simulink model "MiMonza"  (R2023b)
settings: Solver=VariableStepAuto  StartTime=0.0  StopTime=20  MaxStep=0.05
libraries: slpidlib x1
settings Model: Creator=Usuario  LastModifiedBy=Usuario
settings SolverCC: ZeroCrossAlgorithm=Adaptive

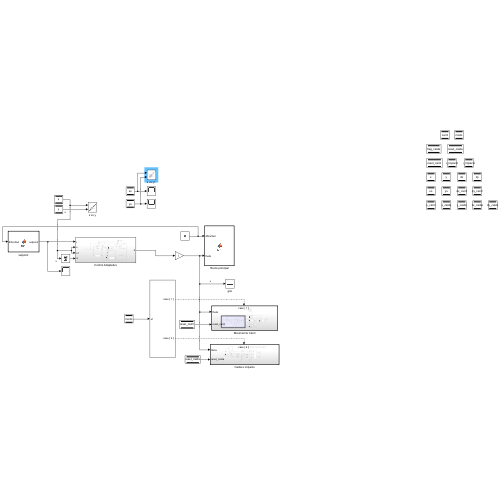
[thumbnail: Simulink's stored preview of the top-level diagram]
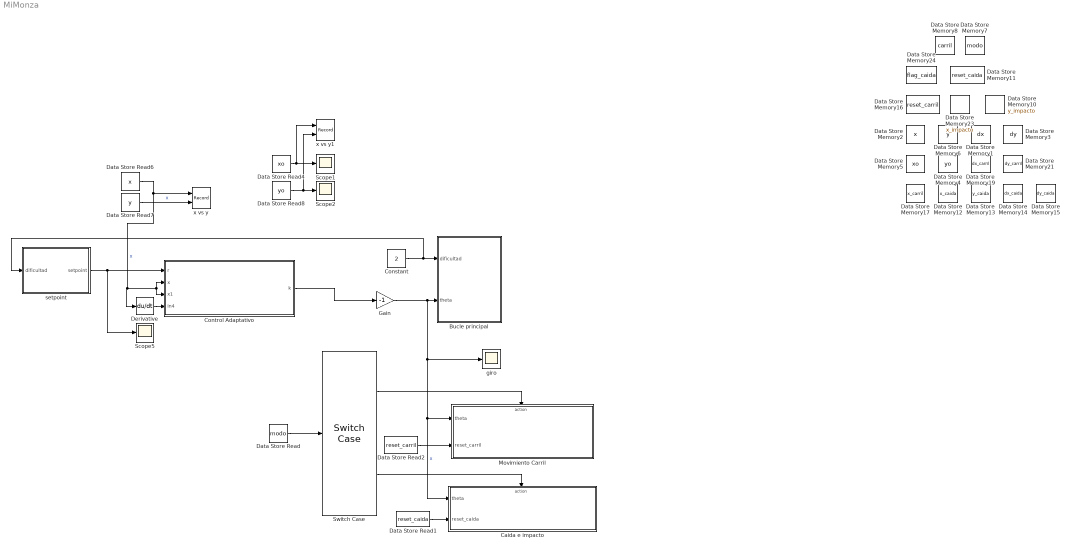
== system MiMonza ==
  " Bucle principal" : MATLAB Function  TreatAsAtomicUnit=on
  Caida e impacto : Subsystem  TreatAsAtomicUnit=on
  Constant : Constant  Value=2
  Control Adaptativo : Subsystem
  Data Store Memory1 : DataStoreMemory  DataStoreName=dx  ReadBeforeWriteMsg=warning  WriteAfterWriteMsg=warning  WriteAfterReadMsg=warning  ShowAdditionalParam=off  OutDataTypeStr=double
  Data Store Memory10 : DataStoreMemory  DataStoreName=y_impacto  ReadBeforeWriteMsg=warning  WriteAfterWriteMsg=warning  WriteAfterReadMsg=warning  ShowAdditionalParam=off  OutDataTypeStr=double
  Data Store Memory11 : DataStoreMemory  DataStoreName=reset_caida  ReadBeforeWriteMsg=warning  WriteAfterWriteMsg=warning  WriteAfterReadMsg=warning  ShowAdditionalParam=off  OutDataTypeStr=double
  Data Store Memory12 : DataStoreMemory  DataStoreName=x_caida  ReadBeforeWriteMsg=warning  WriteAfterWriteMsg=warning  WriteAfterReadMsg=warning  ShowAdditionalParam=off  OutDataTypeStr=double
  Data Store Memory13 : DataStoreMemory  DataStoreName=y_caida  ReadBeforeWriteMsg=warning  WriteAfterWriteMsg=warning  WriteAfterReadMsg=warning  ShowAdditionalParam=off  OutDataTypeStr=double
  Data Store Memory14 : DataStoreMemory  DataStoreName=dx_caida  ReadBeforeWriteMsg=warning  WriteAfterWriteMsg=warning  WriteAfterReadMsg=warning  ShowAdditionalParam=off  OutDataTypeStr=double
  Data Store Memory15 : DataStoreMemory  DataStoreName=dy_caida  ReadBeforeWriteMsg=warning  WriteAfterWriteMsg=warning  WriteAfterReadMsg=warning  ShowAdditionalParam=off  OutDataTypeStr=double
  Data Store Memory16 : DataStoreMemory  DataStoreName=reset_carril  ReadBeforeWriteMsg=warning  WriteAfterWriteMsg=warning  WriteAfterReadMsg=warning  ShowAdditionalParam=off  OutDataTypeStr=double
  Data Store Memory17 : DataStoreMemory  DataStoreName=x_carril  ReadBeforeWriteMsg=warning  WriteAfterWriteMsg=warning  WriteAfterReadMsg=warning  InitialValue=-0.11  ShowAdditionalParam=off  OutDataTypeStr=double
  Data Store Memory19 : DataStoreMemory  DataStoreName=dx_carril  ReadBeforeWriteMsg=warning  WriteAfterWriteMsg=warning  WriteAfterReadMsg=warning  ShowAdditionalParam=off  OutDataTypeStr=double
  Data Store Memory2 : DataStoreMemory  DataStoreName=x  ReadBeforeWriteMsg=warning  WriteAfterWriteMsg=warning  WriteAfterReadMsg=warning  InitialValue=-0.11  ShowAdditionalParam=off  OutDataTypeStr=double
  Data Store Memory21 : DataStoreMemory  DataStoreName=dy_carril  ReadBeforeWriteMsg=warning  WriteAfterWriteMsg=warning  WriteAfterReadMsg=warning  ShowAdditionalParam=off  OutDataTypeStr=double
  Data Store Memory23 : DataStoreMemory  DataStoreName=x_impacto  ReadBeforeWriteMsg=warning  WriteAfterWriteMsg=warning  WriteAfterReadMsg=warning  ShowAdditionalParam=off  OutDataTypeStr=double
  Data Store Memory24 : DataStoreMemory  DataStoreName=flag_caida  ReadBeforeWriteMsg=warning  WriteAfterWriteMsg=warning  WriteAfterReadMsg=warning  ShowAdditionalParam=off  OutDataTypeStr=double
  Data Store Memory3 : DataStoreMemory  DataStoreName=dy  ReadBeforeWriteMsg=warning  WriteAfterWriteMsg=warning  WriteAfterReadMsg=warning  ShowAdditionalParam=off  OutDataTypeStr=double
  Data Store Memory4 : DataStoreMemory  DataStoreName=yo  ReadBeforeWriteMsg=warning  WriteAfterWriteMsg=warning  WriteAfterReadMsg=warning  InitialValue=0.1092  ShowAdditionalParam=off  OutDataTypeStr=double
  Data Store Memory5 : DataStoreMemory  DataStoreName=xo  ReadBeforeWriteMsg=warning  WriteAfterWriteMsg=warning  WriteAfterReadMsg=warning  InitialValue=-0.1  ShowAdditionalParam=off  OutDataTypeStr=double
  Data Store Memory6 : DataStoreMemory  DataStoreName=y  ReadBeforeWriteMsg=warning  WriteAfterWriteMsg=warning  WriteAfterReadMsg=warning  InitialValue=0.106  ShowAdditionalParam=off  OutDataTypeStr=double
  Data Store Memory7 : DataStoreMemory  DataStoreName=modo  ReadBeforeWriteMsg=warning  WriteAfterWriteMsg=warning  WriteAfterReadMsg=warning  InitialValue=1  ShowAdditionalParam=off  OutDataTypeStr=double
  Data Store Memory8 : DataStoreMemory  DataStoreName=carril  ReadBeforeWriteMsg=warning  WriteAfterWriteMsg=warning  WriteAfterReadMsg=warning  InitialValue=1  ShowAdditionalParam=off  OutDataTypeStr=double
  Data Store Read : DataStoreRead  DataStoreName=modo  IndexOptions=Index vector (dialog)  Indices=1  OutputSizes=1
  Data Store Read1 : DataStoreRead  DataStoreName=reset_caida  IndexOptions=Index vector (dialog)  Indices=1  OutputSizes=1
  Data Store Read2 : DataStoreRead  DataStoreName=reset_carril  IndexOptions=Index vector (dialog)  Indices=1  OutputSizes=1
  Data Store Read4 : DataStoreRead  DataStoreName=xo  IndexOptions=Index vector (dialog)  Indices=1  OutputSizes=1
  Data Store Read6 : DataStoreRead  DataStoreName=x  IndexOptions=Index vector (dialog)  Indices=1  OutputSizes=1
  Data Store Read7 : DataStoreRead  DataStoreName=y  IndexOptions=Index vector (dialog)  Indices=1  OutputSizes=1
  Data Store Read8 : DataStoreRead  DataStoreName=yo  IndexOptions=Index vector (dialog)  Indices=1  OutputSizes=1
  Derivative : Derivative
  Gain : Gain  Gain=-1
  Movimiento Carril : Subsystem  TreatAsAtomicUnit=on
  Scope1 : Scope
  Scope2 : Scope
  Scope5 : Scope
  Switch Case : SwitchCase  CaseConditions={1,2}  ShowDefaultCase=off
  giro : Scope
  setpoint : MATLAB Function  TreatAsAtomicUnit=on
  x vs y : Record  FileSettingsInternal="{\"entries\":[{\"content\":{\"excelSettings\":{\"content\":{},\"type\":\"Streamout.ExcelSettings\"}},\"type\":\"Streamout.FileSettingStorage\",\"uuid\":\"\"}],\"packageUris\":[\"http:\\/\\/schema.mathworks.com\\/mf0\\/streamout_blocks\\/R2020a\"],\"version\":\"1.0\"}"  Layout=[1 1]  SignalsInternal="{\"entries\":[{\"content\":{\"signals\":[{\"content\":{\"blockPath\":[],\"dimensions\":[1],\"domain\":\"\",\"lineColor\":\"#a2142f\",\"plots\":[1],\"port\":1,\"sid\":[\"\"],\"signalID\":25020,\"signalName\":\"x\"},\"type\":\"RecordBlkView.Signal\",\"uuid\":\"\"},{\"content\":{\"blockPath\":[],\"dimensions\":[1],\"domain\":\"\",\"lineColor\":\"#139fff\",\"plots\":[1],\"port\":2,\"sid\":[\"\"],\"signalID\":25024,\"signalName\":\"x\"},\"type\":\"RecordBlkView.Signal\",\"uuid\":\"\"}]},\"type\":\"RecordBlkView.InputSignals\",\"uuid\":\"\"}],\"packageUris\":[\"http:\\/\\/schema.mathworks.com\\/mf0\\/streamout_blocks\\/R2020a\"],\"version\":\"1.0\"}"  VisualizationBindings="{\"xyplotplugin\":{\"info\":[{\"series\":[{\"bindingParametersList\":[{\"parameter\":\"X-Axis\",\"signalID\":25020,\"signalName\":\"x\"},{\"parameter\":\"Y-Axis\",\"signalID\":25024,\"signalName\":\"x\"}],\"seriesID\":13625}],\"subplotID\":1}]}}"  CompatibilityTag=XY  st=-1
  x vs y1 : Record  FileSettingsInternal="{\"entries\":[{\"content\":{\"excelSettings\":{\"content\":{},\"type\":\"Streamout.ExcelSettings\"}},\"type\":\"Streamout.FileSettingStorage\",\"uuid\":\"\"}],\"packageUris\":[\"http:\\/\\/schema.mathworks.com\\/mf0\\/streamout_blocks\\/R2020a\"],\"version\":\"1.0\"}"  Layout=[1 1]  SignalsInternal="{\"entries\":[{\"content\":{\"signals\":[{\"content\":{\"blockPath\":[],\"dimensions\":[1],\"domain\":\"\",\"lineColor\":\"#a2142f\",\"plots\":[1],\"port\":1,\"sid\":[\"\"],\"signalID\":25028,\"signalName\":\"Data Store\\nRead4\"},\"type\":\"RecordBlkView.Signal\",\"uuid\":\"\"},{\"content\":{\"blockPath\":[],\"dimensions\":[1],\"domain\":\"\",\"lineColor\":\"#139fff\",\"plots\":[1],\"port\":2,\"sid\":[\"\"],\"signalID\":25032,\"signalName\":\"Data Store\\nRead8\"},\"type\":\"RecordBlkView.Signal\",\"uuid\":\"\"}]},\"type\":\"RecordBlkView.InputSignals\",\"uuid\":\"\"}],\"packageUris\":[\"http:\\/\\/schema.mathworks.com\\/mf0\\/streamout_blocks\\/R2020a\"],\"version\":\"1.0\"}"  VisualizationBindings="{\"xyplotplugin\":{\"info\":[{\"series\":[{\"bindingParametersList\":[{\"parameter\":\"X-Axis\",\"signalID\":25028,\"signalName\":\"Data Store\\nRead4\"},{\"parameter\":\"Y-Axis\",\"signalID\":25032,\"signalName\":\"Data Store\\nRead8\"}],\"seriesID\":36668}],\"subplotID\":1}]}}"  CompatibilityTag=XY  st=-1
  wires:
  Data Store Read2/1 -> Movimiento Carril/2(reset_carril)
  Data Store Read4/1 -> x vs y1/1, Scope1/1
  Data Store Read6/1 -> Derivative/1, Control Adaptativo/2(x), Control Adaptativo/3(x1), x vs y/1  "x"
  Data Store Read/1 -> Switch Case/1
  Gain/1 -> " Bucle principal"/2(theta), Caida e impacto/1(theta), Movimiento Carril/1(theta), giro/1  "x"
  Data Store Read7/1 -> x vs y/2  "x"
  Switch Case/1 -> Movimiento Carril/Action
  Constant/1 -> setpoint/1(dificultad), " Bucle principal"/1(dificultad)
  Data Store Read8/1 -> x vs y1/2, Scope2/1
  setpoint/1(setpoint) -> Control Adaptativo/1(r), Scope5/1
  Switch Case/2 -> Caida e impacto/Action
  Data Store Read1/1 -> Caida e impacto/2(reset_caida)
  Derivative/1 -> Control Adaptativo/4(In4)
  Control Adaptativo/1(k) -> Gain/1

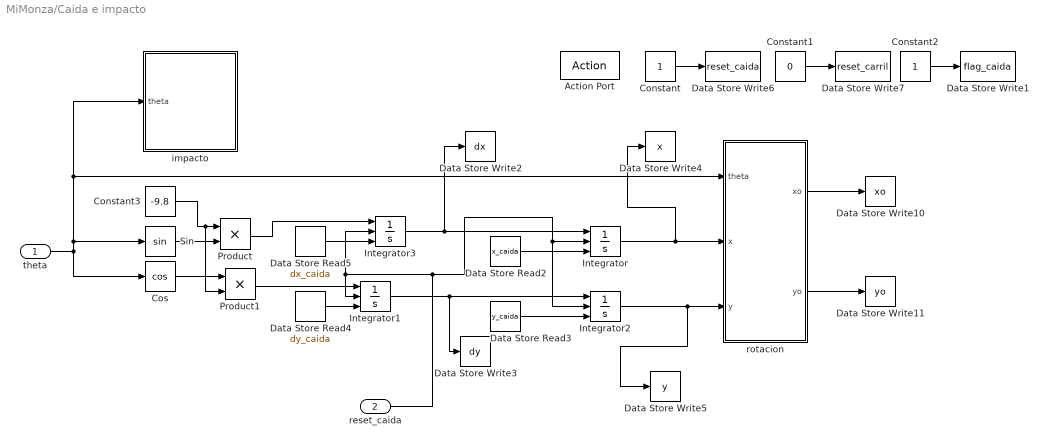
== system MiMonza/Caida e impacto ==
  theta : Inport
  reset_caida : Inport  Port=2
  Action Port : ActionPort  ActionPortLabel=case [ 2 ]:
  Constant : Constant
  Constant1 : Constant  Value=0
  Constant2 : Constant
  Constant3 : Constant  Value=-9.8
  Cos : Trigonometry  Operator=cos
  Data Store Read2 : DataStoreRead  DataStoreName=x_caida  IndexOptions=Index vector (dialog)  Indices=1  OutputSizes=1
  Data Store Read3 : DataStoreRead  DataStoreName=y_caida  IndexOptions=Index vector (dialog)  Indices=1  OutputSizes=1
  Data Store Read4 : DataStoreRead  DataStoreName=dy_caida  IndexOptions=Index vector (dialog)  Indices=1  OutputSizes=1
  Data Store Read5 : DataStoreRead  DataStoreName=dx_caida  IndexOptions=Index vector (dialog)  Indices=1  OutputSizes=1
  Data Store Write1 : DataStoreWrite  DataStoreName=flag_caida  IndexOptions=Index vector (dialog)  Indices=1  OutputSizes=1
  Data Store Write10 : DataStoreWrite  DataStoreName=xo  IndexOptions=Index vector (dialog)  Indices=1  OutputSizes=1
  Data Store Write11 : DataStoreWrite  DataStoreName=yo  IndexOptions=Index vector (dialog)  Indices=1  OutputSizes=1
  Data Store Write2 : DataStoreWrite  DataStoreName=dx  IndexOptions=Index vector (dialog)  Indices=1  OutputSizes=1
  Data Store Write3 : DataStoreWrite  DataStoreName=dy  IndexOptions=Index vector (dialog)  Indices=1  OutputSizes=1
  Data Store Write4 : DataStoreWrite  DataStoreName=x  IndexOptions=Index vector (dialog)  Indices=1  OutputSizes=1
  Data Store Write5 : DataStoreWrite  DataStoreName=y  IndexOptions=Index vector (dialog)  Indices=1  OutputSizes=1
  Data Store Write6 : DataStoreWrite  DataStoreName=reset_caida  IndexOptions=Index vector (dialog)  Indices=1  OutputSizes=1
  Data Store Write7 : DataStoreWrite  DataStoreName=reset_carril  IndexOptions=Index vector (dialog)  Indices=1  OutputSizes=1
  Integrator{,1..3} (4 alike) : Integrator  ExternalReset=falling  InitialConditionSource=external
  Product : Product
  Product1 : Product
  Sin : Trigonometry
  impacto : MATLAB Function  TreatAsAtomicUnit=on
  rotacion : MATLAB Function  TreatAsAtomicUnit=on
  wires:
  Integrator3/1 -> Integrator/1, Data Store Write2/1
  Integrator1/1 -> Integrator2/1, Data Store Write3/1
  Integrator/1 -> Data Store Write4/1, rotacion/2(x)
  Integrator2/1 -> rotacion/3(y), Data Store Write5/1
  reset_caida/1 -> Integrator2/2, Integrator/2, Integrator3/2, Integrator1/2
  Data Store Read4/1 -> Integrator1/3
  Data Store Read5/1 -> Integrator3/3
  Data Store Read2/1 -> Integrator/3
  Data Store Read3/1 -> Integrator2/3
  Constant/1 -> Data Store Write6/1
  Constant1/1 -> Data Store Write7/1
  theta/1 -> Sin/1, rotacion/1(theta), impacto/1(theta), Cos/1
  rotacion/1(xo) -> Data Store Write10/1
  rotacion/2(yo) -> Data Store Write11/1
  Constant2/1 -> Data Store Write1/1
  Product/1 -> Integrator3/1
  Product1/1 -> Integrator1/1
  Cos/1 -> Product1/1
  Sin/1 -> Product/2
  Constant3/1 -> Product1/2, Product/1

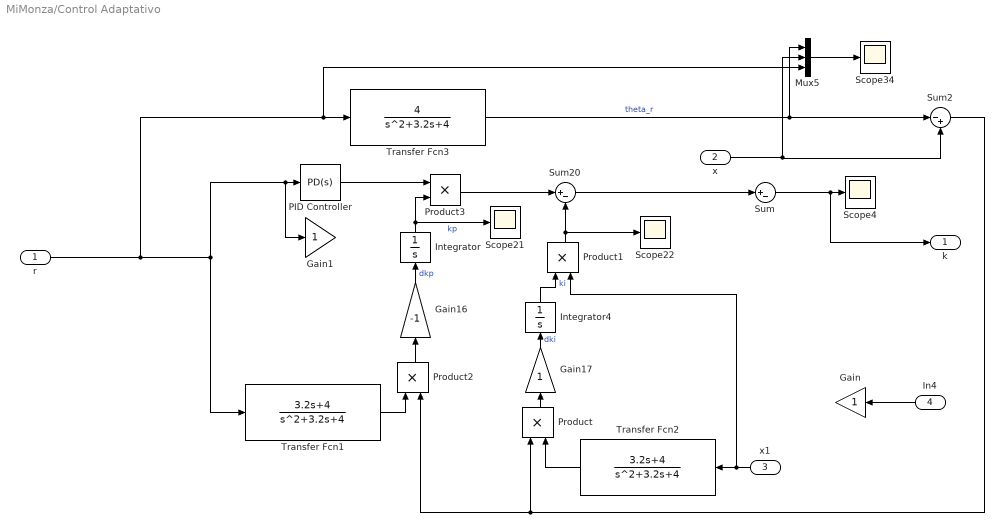
== system MiMonza/Control Adaptativo ==
  r : Inport
  x : Inport  Port=2
  x1 : Inport  Port=3
  In4 : Inport  Port=4
  Gain : Gain
  Gain1 : Gain
  Gain16 : Gain  Gain=-1
  Gain17 : Gain
  Integrator : Integrator  InitialCondition=1
  Integrator4 : Integrator  InitialCondition=1
  Mux5 : Mux  Inputs=3
  PID Controller : slpidlib/PID Controller  Controller=PD  Form=Parallel  TimeDomain=Continuous-time  UseExternalTs=off  SampleTime=-1  IntegratorMethod=Forward Euler  FilterMethod=Forward Euler  ControllerParametersSource=internal  P=0.2  I=1  UseKiTs=off  D=0.05  N=10  UseFilter=on  TunerSelectOption=Transfer Function Based (PID Tuner App)  InitialConditionSource=internal  InitialConditionForIntegrator=0  InitialConditionForFilter=0  DifferentiatorICPrevScaledInput=0  ExternalReset=none  TrackingMode=off  Kt=1  LimitOutput=off  SatLimitsSource=internal  UpperSaturationLimit=inf  LowerSaturationLimit=-inf  LinearizeAsGain=on  AntiWindupMode=none  Kb=1  LimitIntegrator=off  UpperIntegratorSaturationLimit=inf  LowerIntegratorSaturationLimit=-inf  POutMin=[]  POutMax=[]  IOutMin=[]  IOutMax=[]  DOutMin=[]  DOutMax=[]  NOutMin=[]  NOutMax=[]  SumOutMin=[]  SumOutMax=[]  SaturationOutMin=[]  SaturationOutMax=[]  PParamMin=[]  PParamMax=[]  IParamMin=[]  IParamMax=[]  DParamMin=[]  DParamMax=[]  NParamMin=[]  NParamMax=[]  KbParamMin=[]  KbParamMax=[]  KtParamMin=[]  KtParamMax=[]  KbOutMin=[]  KbOutMax=[]  KtOutMin=[]  KtOutMax=[]  IntegratorOutMin=[]  IntegratorOutMax=[]  FilterOutMin=[]  FilterOutMax=[]  SumI1OutMin=[]  SumI1OutMax=[]  SumI2OutMin=[]  SumI2OutMax=[]  SumI3OutMin=[]  SumI3OutMax=[]  SumI4OutMin=[]  SumI4OutMax=[]  SumDOutMin=[]  SumDOutMax=[]  DifferentiatorOutMin=[]  DifferentiatorOutMax=[]  FilterDiffOutCoefMin=[]  FilterDiffOutCoefMax=[]  ReciprocalOutMin=[]  ReciprocalOutMax=[]  SumDenOutMin=[]  SumDenOutMax=[]  SumNumOutMin=[]  SumNumOutMax=[]  DivideOutMin=[]  DivideOutMax=[]  UdiffTsProdOutMin=[]  UdiffTsProdOutMax=[]  NTsProdOutMin=[]  NTsProdOutMax=[]  UintegralTsProdOutMin=[]  UintegralTsProdOutMax=[]  UngainTsProdOutMin=[]  UngainTsProdOutMax=[]  ClampingZeroOutDataTypeStr=Inherit: Inherit via back propagation  ClampingZeroOutMin=[]  ClampingZeroOutMax=[]  FilterDenConstantOutDataTypeStr=Inherit: Inherit via back propagation  FilterDenConstantOutMin=[]  FilterDenConstantOutMax=[]  PCopyOutDataTypeStr=Inherit: Inherit via back propagation  PCopyOutMin=[]  PCopyOutMax=[]  NCopyOutDataTypeStr=Inherit: Inherit via back propagation  NCopyOutMin=[]  NCopyOutMax=[]  IntegratorContinuousStateAttributes=''  IntegratorStateMustResolveToSignalObject=off  IntegratorRTWStateStorageClass=Auto  FilterContinuousStateAttributes=''  FilterStateMustResolveToSignalObject=off  FilterRTWStateStorageClass=Auto  ParallelPVariant=InternalParameters  IdealPVariant=Disabled  IVariant=Disabled  DVariant=InternalParameters  IntegratorVariant=Disabled  SatVariant=Disabled  AWVariant=Disabled  PCopyVariant=Disabled  TRVariant=Disabled  FdbkBlocksVariant=Forward  IdealPFdbkVariant=Disabled  SatFdbkVariant=Disabled  DerivativeFilterVariant=ContFilter  NVariant=InternalParameters  NCopyVariant=Disabled  FilterICVariant=InternalICsFilter  IntegratorICVariant=Disabled  ExternalResetVariant=Disabled  TRSumVariant=Passthrough  SumFdbkVariant=Disabled  SumVariant=Sum_PD  TsampFilterVariant=InternalTs  TsampNgainVariant=Passthrough  TsampIntegralVariant=Disabled_SignalSpec  ExternalSaturationOutDataTypeStr=Inherit: Same as second input
  Product{,1..3} (4 alike) : Product
  Scope{4,21..22,34} (4 alike) : Scope
  Sum : Sum  Inputs=|+-
  Sum2 : Sum  Inputs=|-+
  Sum20 : Sum  Inputs=|+-
  Transfer Fcn1 : TransferFcn  Numerator=[3.2 4]  Denominator=[1 3.2 4]
  Transfer Fcn2 : TransferFcn  Numerator=[3.2 4]  Denominator=[1 3.2 4]
  Transfer Fcn3 : TransferFcn  Numerator=[4]  Denominator=[1 3.2 4]
  k : Outport
  wires:
  r/1 -> Transfer Fcn3/1, Mux5/3, Transfer Fcn1/1, Gain1/1, PID Controller/1
  x1/1 -> Transfer Fcn2/1, Product1/2
  x/1 -> Mux5/2, Sum2/2
  Product1/1 -> Sum20/2, Scope22/1
  Gain16/1 -> Integrator/1  "dkp"
  Mux5/1 -> Scope34/1
  Product3/1 -> Sum20/1
  Transfer Fcn3/1 -> Mux5/1, Sum2/1  "theta_r"
  Product2/1 -> Gain16/1
  Integrator/1 -> Product3/2, Scope21/1  "kp"
  Integrator4/1 -> Product1/1  "ki"
  Transfer Fcn1/1 -> Product2/1
  Product/1 -> Gain17/1
  Gain17/1 -> Integrator4/1  "dki"
  Sum/1 -> k/1, Scope4/1
  Transfer Fcn2/1 -> Product/2
  Sum20/1 -> Sum/1
  Sum2/1 -> Product/1, Product2/2
  In4/1 -> Gain/1
  PID Controller/1 -> Product3/1

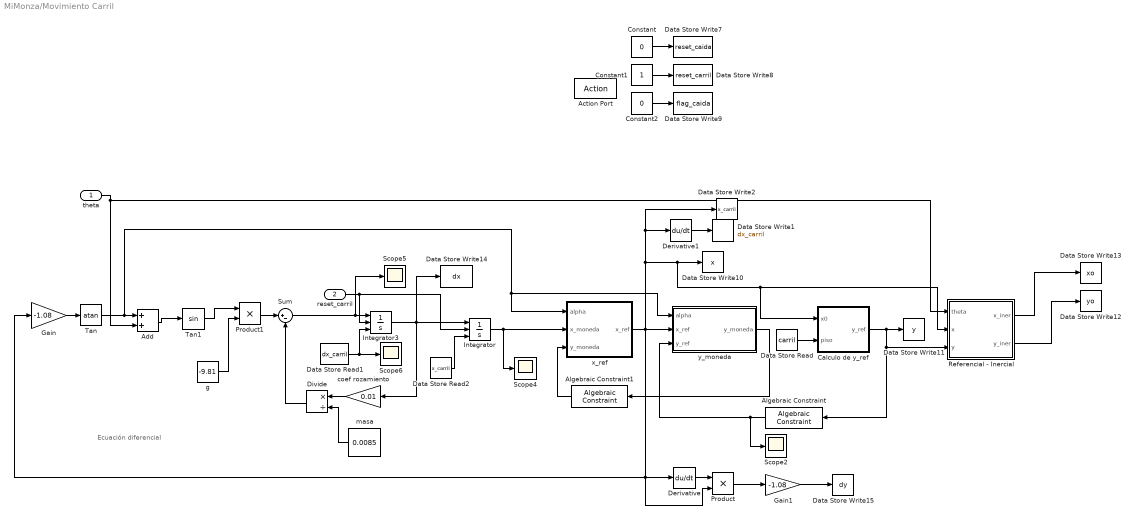
== system MiMonza/Movimiento Carril ==
  note: Ecuación diferencial
  theta : Inport
  reset_carril : Inport  Port=2
  Action Port : ActionPort  ActionPortLabel=case [ 1 ]:
  Add : Sum
  Algebraic Constraint : AlgebraicConstraint  Constraint=f(z) = z
  Algebraic Constraint1 : AlgebraicConstraint  Constraint=f(z) = z
  Calculo de y_ref : MATLAB Function  TreatAsAtomicUnit=on
  Constant : Constant  Value=0
  Constant1 : Constant
  Constant2 : Constant  Value=0
  Data Store Read : DataStoreRead  DataStoreName=carril  IndexOptions=Index vector (dialog)  Indices=1  OutputSizes=1
  Data Store Read1 : DataStoreRead  DataStoreName=dx_carril  IndexOptions=Index vector (dialog)  Indices=1  OutputSizes=1
  Data Store Read2 : DataStoreRead  DataStoreName=x_carril  IndexOptions=Index vector (dialog)  Indices=1  OutputSizes=1
  Data Store Write1 : DataStoreWrite  DataStoreName=dx_carril  IndexOptions=Index vector (dialog)  Indices=1  OutputSizes=1
  Data Store Write10 : DataStoreWrite  DataStoreName=x  IndexOptions=Index vector (dialog)  Indices=1  OutputSizes=1
  Data Store Write11 : DataStoreWrite  DataStoreName=y  IndexOptions=Index vector (dialog)  Indices=1  OutputSizes=1
  Data Store Write12 : DataStoreWrite  DataStoreName=yo  IndexOptions=Index vector (dialog)  Indices=1  OutputSizes=1
  Data Store Write13 : DataStoreWrite  DataStoreName=xo  IndexOptions=Index vector (dialog)  Indices=1  OutputSizes=1
  Data Store Write14 : DataStoreWrite  DataStoreName=dx  IndexOptions=Index vector (dialog)  Indices=1  OutputSizes=1
  Data Store Write15 : DataStoreWrite  DataStoreName=dy  IndexOptions=Index vector (dialog)  Indices=1  OutputSizes=1
  Data Store Write2 : DataStoreWrite  DataStoreName=x_carril  IndexOptions=Index vector (dialog)  Indices=1  OutputSizes=1
  Data Store Write7 : DataStoreWrite  DataStoreName=reset_caida  IndexOptions=Index vector (dialog)  Indices=1  OutputSizes=1
  Data Store Write8 : DataStoreWrite  DataStoreName=reset_carril  IndexOptions=Index vector (dialog)  Indices=1  OutputSizes=1
  Data Store Write9 : DataStoreWrite  DataStoreName=flag_caida  IndexOptions=Index vector (dialog)  Indices=1  OutputSizes=1
  Derivative : Derivative
  Derivative1 : Derivative
  Divide : Product  Inputs=*/
  Gain : Gain  Gain=-1.08
  Gain1 : Gain  Gain=-1.08
  Integrator : Integrator  ExternalReset=falling  InitialConditionSource=external
  Integrator3 : Integrator  ExternalReset=falling  InitialConditionSource=external
  Product : Product
  Product1 : Product
  Referencial - Inercial : MATLAB Function  TreatAsAtomicUnit=on
  Scope{2,4..6} (4 alike) : Scope
  Sum : Sum  Inputs=|+-
  Tan : Trigonometry  Operator=atan
  Tan1 : Trigonometry
  coef rozamiento : Gain  Gain=0.01
  g : Constant  Value=-9.81
  masa : Constant  Value=0.0085
  x_ref : MATLAB Function  TreatAsAtomicUnit=on
  y_moneda : MATLAB Function  TreatAsAtomicUnit=on
  wires:
  Constant/1 -> Data Store Write7/1
  Constant1/1 -> Data Store Write8/1
  Constant2/1 -> Data Store Write9/1
  reset_carril/1 -> Integrator3/2, Integrator/2
  Algebraic Constraint/1 -> y_moneda/3(y_ref), Scope2/1
  Tan/1 -> Add/1, y_moneda/1(alpha), x_ref/1(alpha)
  Tan1/1 -> Product1/1
  Integrator/1 -> Scope4/1, x_ref/2(x_moneda)
  Product1/1 -> Sum/1
  Referencial - Inercial/2(y_iner) -> Data Store Write12/1
  Gain/1 -> Tan/1
  Data Store Read2/1 -> Integrator/3
  Sum/1 -> Scope5/1, Integrator3/1
  Data Store Read1/1 -> Scope6/1, Integrator3/3
  theta/1 -> Add/2, Referencial - Inercial/1(theta)
  Integrator3/1 -> coef rozamiento/1, Data Store Write14/1, Integrator/1
  Calculo de y_ref/1(y_ref) -> Algebraic Constraint/1, Referencial - Inercial/3(y), Data Store Write11/1
  Referencial - Inercial/1(x_iner) -> Data Store Write13/1
  Data Store Read/1 -> Calculo de y_ref/2(piso)
  g/1 -> Product1/2
  Divide/1 -> Sum/2
  Add/1 -> Tan1/1
  Derivative/1 -> Product/1
  Product/1 -> Gain1/1
  Gain1/1 -> Data Store Write15/1
  x_ref/1(x_ref) -> Gain/1, Product/2, Derivative/1, Data Store Write2/1, Derivative1/1, Calculo de y_ref/1(x0), Referencial - Inercial/2(x), Data Store Write10/1, y_moneda/2(x_ref)
  y_moneda/1(y_moneda) -> Algebraic Constraint1/1
  Algebraic Constraint1/1 -> x_ref/3(y_moneda)
  coef rozamiento/1 -> Divide/1
  masa/1 -> Divide/2
  Derivative1/1 -> Data Store Write1/1

== matlab function MiMonza/Caida e impacto/rotacion ==
  data: xo output; yo output; theta input; x input; y input
function [xo,yo] = fcn(theta,x,y)
xo=x*cos(theta)-y*sin(theta);
yo=x*sin(theta)+y*cos(theta);
end

== matlab function MiMonza/Movimiento Carril/Calculo de y_ref ==
  data: x0 input; y_ref output; piso input
function y_ref  = fcn(x0, piso)

switch piso
    case 1
        y_ref= -0.54*x0^2 + 0.1143;
    case 2
        y_ref= -0.54*x0^2 + 0.0686;
    case 3
        y_ref= -0.54*x0^2 + 0.03;
    case 4
        y_ref= -0.54*x0^2 - 0.03;  
    case 5
        y_ref= -0.54*x0^2 - 0.0686; 
    case 6
        y_ref= -0.54*x0^2 - 0.1143;
    case 7
        y_ref= -0.54*x0^2 - 0.16;
    otherwise
        y_ref = 0;
end

== matlab function MiMonza/Movimiento Carril/x_ref ==
  settings: updateMethod=DISCRETE
  data: alpha input; x_ref output; x_moneda input; y_moneda input
function x_ref  = rotate(alpha,x_moneda,y_moneda)
x_ref =  x_moneda*cos(alpha)-y_moneda*sin(alpha);

== matlab function MiMonza/Movimiento Carril/Referencial - Inercial ==
  settings: updateMethod=DISCRETE
  data: theta input; x_iner output; x input; y input; y_iner output
function [x_iner,y_iner] = rotate(theta,x,y)
x_iner =  x*cos(theta)-y*sin(theta);
y_iner = x*sin(theta) + y*cos(theta);

== matlab function MiMonza/setpoint ==
  settings: updateMethod=DISCRETE
  data: setpoint output; carril data_store_memory; x data_store_memory; dificultad input
function setpoint = fcn(dificultad)
coder.extrinsic('finalesRieles');
global carril

%Inicializa finales de riel:
x1derecha = 0;
x2izquierda = 0;
x3derecha = 0;
x4izquierda = 0;
x5derecha = 0; 
x6izquierda = 0;
x7derecha = 0;

%Indicamos el setpoint inicial
setpoint = 0.11;
[x1derecha,x2izquierda,x3derecha,x4izquierda,x5derecha,x6izquierda,x7derecha] = finalesRieles(dificultad);

switch carril

    case 1
        setpoint = x1derecha;
    case 2
        setpoint = x2izquierda;
    case 3
        setpoint = x3derecha;
    case 4
        setpoint = x4izquierda;
    case 5
        setpoint = x5derecha;
    case 6
        setpoint = x6izquierda;
    case 7
        setpoint = x7derecha+0.1;
        
end

%setpoint=setpoint/2;

== matlab function MiMonza/Movimiento Carril/y_moneda ==
  settings: updateMethod=DISCRETE
  data: alpha input; y_moneda output; x_ref input; y_ref input
function y_moneda  = rotate(alpha,x_ref,y_ref)
y_moneda =  -x_ref*sin(alpha)+y_ref*cos(alpha);

== matlab function MiMonza/ Bucle principal ==
  settings: updateMethod=DISCRETE
  data: dificultad input; theta input; x data_store_memory; y data_store_memory; dx data_store_memory; carril data_store_memory; modo data_store_memory; reset_caida data_store_memory; x_caida data_store_memory; y_caida data_store_memory; dx_caida data_store_memory; dy_caida data_store_memory; reset_carril data_store_memory; x_carril data_store_memory; dx_carril data_store_memory; dy data_store_memory; x_impacto data_store_memory; y_impacto data_store_memory; flag_caida data_store_memory; xo data_store_memory; yo data_store_memory
function fcn(dificultad,theta)
coder.extrinsic('gcs');
coder.extrinsic('set_param');
coder.extrinsic('finalesRieles');
global carril
global modo

global x
global y
global xo
global yo
global dx
global dy
global x_caida
global y_caida
global dx_caida
global dy_caida
global x_carril
global dx_carril
global x_impacto
global y_impacto

global reset_carril
global reset_caida
global flag_caida
caida=5;

%Inicialización
x1derecha = 0;
x2izquierda = 0;
x3derecha = 0;
x4izquierda = 0;
x5derecha = 0; 
x6izquierda = 0;
x7derecha = 0;

[x1derecha,x2izquierda,x3derecha,x4izquierda,x5derecha,x6izquierda,x7derecha] = finalesRieles(dificultad);

if modo == 1 %La moneda se mueve por alguno de los carriles
    reset_carril = 1; % Para que cuando se 
    flag_caida = 0;
    
    switch carril   % si entra en alguno de los if, la bola está fuera del carril, por lo que está cayendo
        case 1
            if x >= x1derecha 
                modo = 2;
                caida = 0;
                reset_caida = 0;
            end
        case 2
            if x <= x2izquierda
                modo = 2;
                caida = 0;
                reset_caida = 0;                
            end
        case 3
            if x >= x3derecha
                modo = 2;
                caida = 0;
                reset_caida = 0;
            end
        case 4
            if x <= x4izquierda
                modo = 2;
                caida = 0;
                reset_caida = 0;                
            end
        case 5
            if x >= x5derecha
                modo = 2;
                caida = 0;
                reset_caida = 0;
            end
        case 6
            if x <= x6izquierda
                modo = 2;
                caida = 0;
                reset_caida = 0;                
            end
        case 7
            if x >= x7derecha 
                set_param(gcs, 'SimulationCommand', 'stop')
            end
    end
    if caida == 0
        x_caida = x;
        y_caida = y;    
        dx_caida = dx;  
        dy_caida = dy;
    end
elseif modo == 2    
        reset_caida = 1;
        flag_caida = 1;
        if y<=y_impacto
            reset_carril = 0;
            carril = carril + 1;   
            x_carril = x_impacto; 
            dx_carril = dx;
            modo=1;
        end
    end
end

== matlab function MiMonza/Caida e impacto/impacto ==
  settings: updateMethod=DISCRETE
  data: carril data_store_memory; x data_store_memory; y data_store_memory; theta input; dx data_store_memory; dy data_store_memory; x_impacto data_store_memory; y_impacto data_store_memory; x_caida data_store_memory; y_caida data_store_memory; dx_caida data_store_memory; dy_caida data_store_memory; flag_caida data_store_memory
function fcn(theta)


pendiente = -0.54;
global x_impacto
global y_impacto
global dx_caida
global dy_caida
global x_caida
global y_caida
global flag_caida
global carril
x_impacto = 0;
y_impacto = 0;
coder.extrinsic('impacto');
    if flag_caida == 1
        switch carril
            case 1
                altura = 0.0686;
                [x_impacto,y_impacto]=calculo(x_caida,dx_caida,y_caida,dy_caida,altura,pendiente,theta);
            case 2
                altura = 0.03;
                [x_impacto,y_impacto]=calculo(x_caida,dx_caida,y_caida,dy_caida,altura,pendiente,theta);
            case 3
                altura = -0.03;
                [x_impacto,y_impacto]=calculo(x_caida,dx_caida,y_caida,dy_caida,altura,pendiente,theta);
            case 4
                altura = -0.0686;
                [x_impacto,y_impacto]=calculo(x_caida,dx_caida,y_caida,dy_caida,altura,pendiente,theta);
            case 5
                altura = -0.1143;
                [x_impacto,y_impacto]=calculo(x_caida,dx_caida,y_caida,dy_caida,altura,pendiente,theta);
            case 6
                altura = -0.16;
                [x_impacto,y_impacto]=calculo(x_caida,dx_caida,y_caida,dy_caida,altura,pendiente,theta);
        end
    end

end
